simulink model "PID31"  (R2021b)
settings: Solver=VariableStepAuto  StartTime=0.0  StopTime=10.0  RelTol=1e-3
libraries: slpidlib x1
settings Model: Creator=rkhas  LastModifiedBy=rkhas

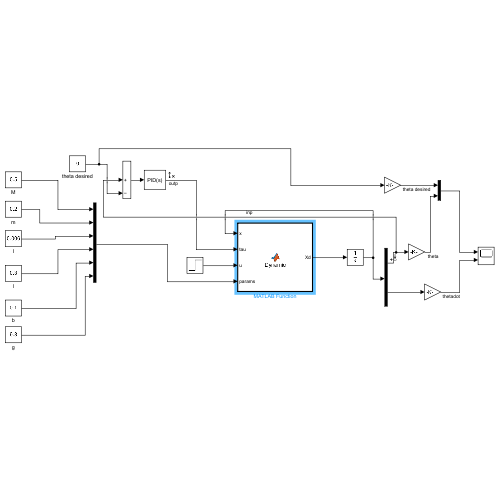
[thumbnail: Simulink's stored preview of the top-level diagram]
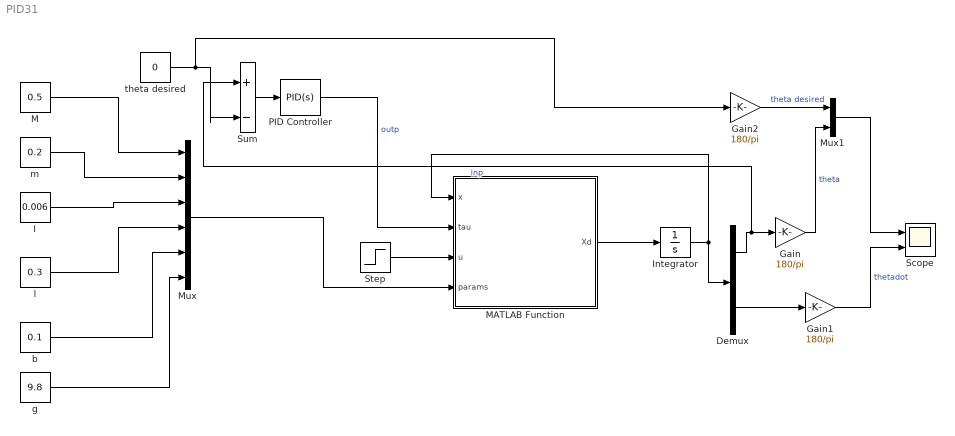
== system PID31 ==
  Demux : Demux  Outputs=2
  Gain : Gain  Gain=180/pi
  Gain1 : Gain  Gain=180/pi
  Gain2 : Gain  Gain=180/pi
  I : Constant  Value=0.006
  Integrator : Integrator  InitialCondition=pi/2
  M : Constant  Value=0.5
  MATLAB Function : MATLAB Function  TreatAsAtomicUnit=on
  Mux : Mux  Inputs=6
  Mux1 : Mux  Inputs=2
  PID Controller : slpidlib/PID Controller  Controller=PID  Form=Parallel  TimeDomain=Continuous-time  UseExternalTs=off  SampleTime=-1  IntegratorMethod=Forward Euler  FilterMethod=Forward Euler  ControllerParametersSource=internal  P=-3.85793370988613  I=-7.28748226385827  D=0.0538073296526276  UseFilter=on  N=11.8940326833611  TunerSelectOption=Transfer Function Based (PID Tuner App)  InitialConditionSource=internal  InitialConditionForIntegrator=0  InitialConditionForFilter=0  DifferentiatorICPrevScaledInput=0  ExternalReset=none  TrackingMode=off  Kt=1  LimitOutput=off  SatLimitsSource=internal  UpperSaturationLimit=inf  LowerSaturationLimit=-inf  LinearizeAsGain=on  AntiWindupMode=none  Kb=1  POutMin=[]  POutMax=[]  IOutMin=[]  IOutMax=[]  DOutMin=[]  DOutMax=[]  NOutMin=[]  NOutMax=[]  SumOutMin=[]  SumOutMax=[]  SaturationOutMin=[]  SaturationOutMax=[]  PParamMin=[]  PParamMax=[]  IParamMin=[]  IParamMax=[]  DParamMin=[]  DParamMax=[]  NParamMin=[]  NParamMax=[]  KbParamMin=[]  KbParamMax=[]  KtParamMin=[]  KtParamMax=[]  KbOutMin=[]  KbOutMax=[]  KtOutMin=[]  KtOutMax=[]  IntegratorOutMin=[]  IntegratorOutMax=[]  FilterOutMin=[]  FilterOutMax=[]  SumI1OutMin=[]  SumI1OutMax=[]  SumI2OutMin=[]  SumI2OutMax=[]  SumI3OutMin=[]  SumI3OutMax=[]  SumI4OutMin=[]  SumI4OutMax=[]  SumDOutMin=[]  SumDOutMax=[]  DifferentiatorOutMin=[]  DifferentiatorOutMax=[]  FilterDiffOutCoefMin=[]  FilterDiffOutCoefMax=[]  ReciprocalOutMin=[]  ReciprocalOutMax=[]  SumDenOutMin=[]  SumDenOutMax=[]  SumNumOutMin=[]  SumNumOutMax=[]  DivideOutMin=[]  DivideOutMax=[]  UdiffTsProdOutMin=[]  UdiffTsProdOutMax=[]  NTsProdOutMin=[]  NTsProdOutMax=[]  UintegralTsProdOutMin=[]  UintegralTsProdOutMax=[]  UngainTsProdOutMin=[]  UngainTsProdOutMax=[]  IntegratorContinuousStateAttributes=''  IntegratorStateMustResolveToSignalObject=off  IntegratorRTWStateStorageClass=Auto  FilterContinuousStateAttributes=''  FilterStateMustResolveToSignalObject=off  FilterRTWStateStorageClass=Auto  ParallelPVariant=InternalParameters  IdealPVariant=Disabled  IVariant=InternalParameters  DVariant=InternalParameters  IntegratorVariant=Continuous  SatVariant=Disabled  AWVariant=Passthrough  PCopyVariant=Disabled  TRVariant=Disabled  FdbkBlocksVariant=Forward  IdealPFdbkVariant=Disabled  SatFdbkVariant=Disabled  DerivativeFilterVariant=ContFilter  NVariant=InternalParameters  NCopyVariant=Disabled  FilterICVariant=InternalICsFilter  IntegratorICVariant=InternalICs  ExternalResetVariant=Disabled  TRSumVariant=Passthrough  SumFdbkVariant=Disabled  SumVariant=Sum_PID  TsampFilterVariant=InternalTs  TsampNgainVariant=Passthrough  TsampIntegralVariant=Passthrough  ExternalSaturationOutDataTypeStr=Inherit: Same as second input
  Scope : Scope  NumInputPorts=2
  Step : Step  SampleTime=0
  Sum : Sum  Inputs=|+-
  b : Constant  Value=0.1
  g : Constant  Value=9.8
  l : Constant  Value=0.3
  m : Constant  Value=0.2
  theta desired : Constant  Value=0
  wires:
  M/1 -> Mux/1
  m/1 -> Mux/2
  I/1 -> Mux/3
  l/1 -> Mux/4
  b/1 -> Mux/5
  g/1 -> Mux/6
  Mux/1 -> MATLAB Function/4(params)
  Step/1 -> MATLAB Function/3(u)
  MATLAB Function/1(Xd) -> Integrator/1
  Integrator/1 -> MATLAB Function/1(x), Demux/1
  Demux/1 -> Sum/1, Gain/1  "inp"
  Demux/2 -> Gain1/1
  Gain1/1 -> Scope/2  "thetadot"
  theta desired/1 -> Gain2/1, Sum/2
  Sum/1 -> PID Controller/1
  PID Controller/1 -> MATLAB Function/2(tau)  "outp"
  Gain2/1 -> Mux1/1  "theta desired"
  Gain/1 -> Mux1/2  "theta"
  Mux1/1 -> Scope/1

== matlab function PID31/MATLAB Function ==
  data: x input; tau input; u input; Xd output; params input
function Xd = Dynamic(x,tau,u,params)
M = params(1);
m = params(2);
b = params(5);
I = params(3);
g = params(6);
l = params(4);
Xd = zeros(2,1);
Xd(2,1) = x(2);
Xd(1,1) = ((m*m*l*l*g)/(I*(M+m)+M*m*l*l))*tau + ((I+m*l*l)/(I*(M+m)+M*m*l*l))*u;
